simulink subsystem "HVDCPassThroughSSC"  (R2024b)
settings: Solver=VariableStepAuto  StartTime=0.0  StopTime=10.0  RelTol=1e-3
undefined symbols (not defined in the file): BattNeg, BattPos, EnvAirTemp, HVDCNeg, HVDCPos
libraries: fl_lib x1
settings Model: ModifiedByFormat=The MathWorks, Inc.  Creator=The MathWorks, Inc.  LastModifiedBy=The MathWorks, Inc.
settings OptimizationCC: ReuseModelBlockBuffer=off
settings RTWCC: GPUComputeCapability=3.5

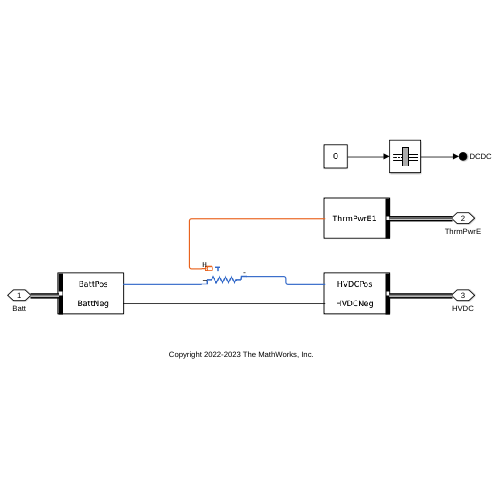
[thumbnail: Simulink's stored preview of the top-level diagram]
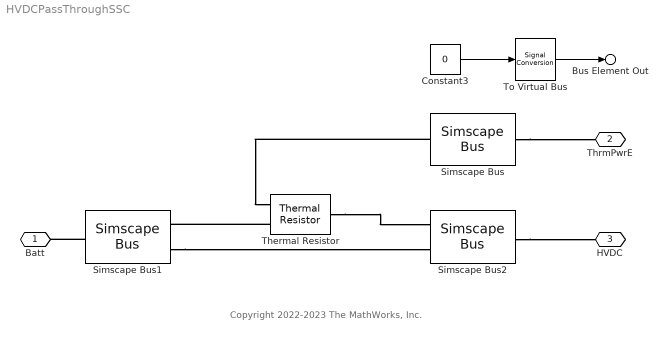
== system HVDCPassThroughSSC ==
  note: Copyright 2022-2023 The MathWorks, Inc.
  Constant3 : Constant  Value=0  OutDataTypeStr=Bus: DCDCBUS  SampleTime=-1
  Simscape Bus : SimscapeBus  HierarchyStrings=ThrmPwrE1
  Simscape Bus1 : SimscapeBus  HierarchyStrings=BattPos;BattNeg
  Simscape Bus2 : SimscapeBus  HierarchyStrings=HVDCPos;HVDCNeg
  Thermal Resistor : fl_lib/Electrical/Electrical Elements/Thermal Resistor  R0=1e-6 Ohm  T0=EnvAirTemp K  alpha=50e-6 1/K  tc=10 s  K_d=1e-3 W/K  T_specify=on  T_priority=High  T=EnvAirTemp K  T_nominal_specify=off  T_nominal_value=1  T_nominal_unit=K
      settings: InternalSimscapePortConfiguration="{\"Bottom\":[],\"Left\":[{\"id\":\"H\",\"label\":\"H\",\"type\":\"foundation.thermal.thermal\"},{\"id\":\"p\",\"label\":\"+\",\"type\":\"foundation.electrical.electrical\"}],\"Right\":[{\"id\":\"n\",\"label\":\"-\",\"type\":\"foundation.electrical.electrical\"}],\"Top\":[]}"
  To Virtual Bus : SignalConversion  ConversionOutput=Virtual bus  OverrideOpt=off
  Batt : PMIOPort  Side=Left
  ThrmPwrE : PMIOPort  Port=2  Side=Right
  HVDC : PMIOPort  Port=3  Side=Right
  Bus Element Out : Outport  PortName=DCDC
  wires:
  Constant3/1 -> To Virtual Bus/1
  To Virtual Bus/1 -> Bus Element Out/1
  connections:
  Simscape Bus/RConn1 -- ThrmPwrE/RConn1
  Simscape Bus/LConn1 -- Thermal Resistor/LConn1
  Thermal Resistor/RConn1 -- Simscape Bus2/LConn1
  Thermal Resistor/LConn2 -- Simscape Bus1/LConn1
  Simscape Bus1/RConn1 -- Batt/RConn1
  Simscape Bus2/RConn1 -- HVDC/RConn1
  Simscape Bus1/LConn2 -- Simscape Bus2/LConn2
